simulink model "NL_guidance"  (R2026a)
settings: Solver=ode15s  StopTime=60  MaxStep=0.05  MinStep=1e-8  AbsTol=1e-4
StartFcn:
  | ins_initial_state_xplane;
values from neighbouring files (symbols this model uses):
  C_alt = evalin('base', 'C_alt')    [gui_waypoints.m]    (also in scr_aux_wp.m)
  C_phi = evalin('base', 'C_phi')    [gui_waypoints.m]    (also in scr_aux_wp.m)
  C_theta = evalin('base', 'C_theta')    [gui_waypoints.m]    (also in scr_aux_wp.m)
  C_vel = evalin('base', 'C_vel')    [gui_waypoints.m]    (also in scr_aux_wp.m)
  Kp = evalin('base', 'Kp')    [gui_waypoints.m]    (also in inicializar.m = 0.119; scr_aux_wp.m)
  Kq = evalin('base', 'Kq')    [gui_waypoints.m]    (also in inicializar.m = 0.1; scr_aux_wp.m)
  Kr = evalin('base', 'Kr')    [gui_waypoints.m]    (also in inicializar.m = 0.15; scr_aux_wp.m)
  R_accept = 80    [inicializar.m]    (also in scr_waypoints.m)
  TrimInput = evalin('base', 'TrimInput')    [gui_waypoints.m]    (also in inicializar.m = Ue'; scr_aux_wp.m)
  WPs = [ ... (first row only)    [inicializar.m]
  Xe = evalin('base', 'Xe')    [gui_waypoints.m]    (also in scr_aux_wp.m)
undefined symbols (not defined in the file or in its folder): sensors
libraries: slpidlib x5
settings Model: Creator=anade  LastModifiedBy=julio
settings DataIOCC: SaveState=on

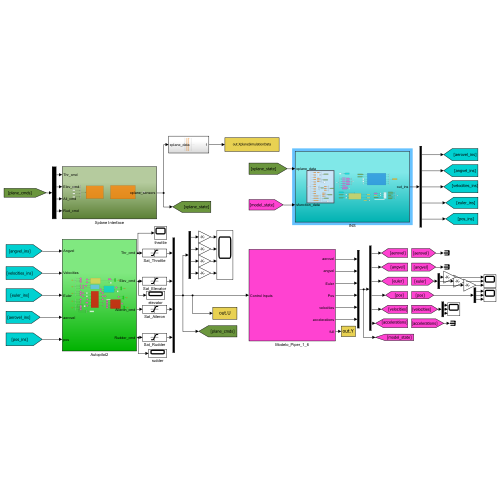
[thumbnail: Simulink's stored preview of the top-level diagram]
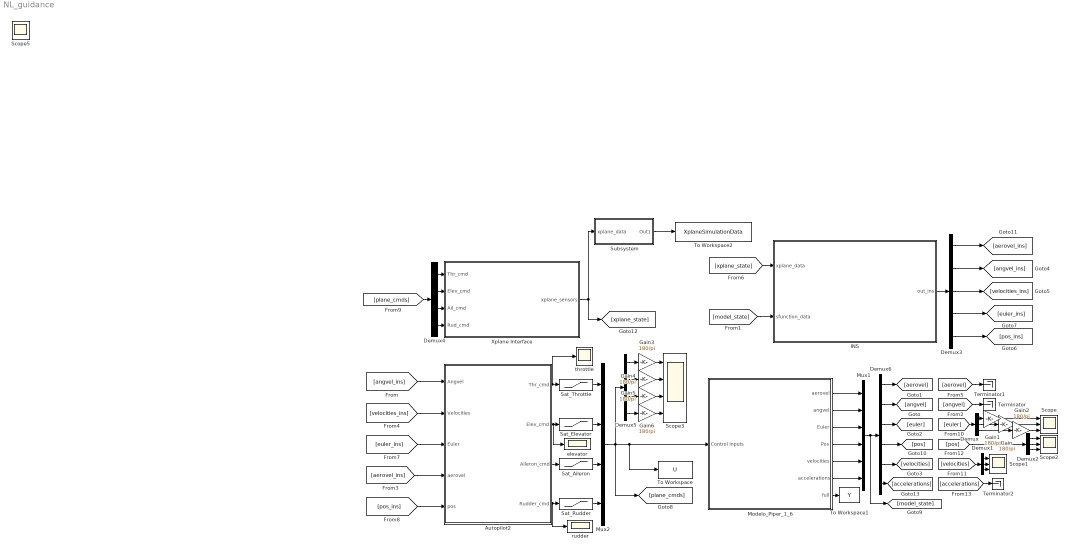
== system NL_guidance ==
  Autopilot2 : Subsystem
  Demux : Demux  Outputs=3
  Demux1 : Demux  Outputs=3
  Demux2 : Demux  Outputs=3
  Demux3 : Demux  Outputs=5
  Demux4 : Demux
  Demux5 : Demux
  Demux6 : Demux  Outputs=6
  Gain{,1..6} (7 alike) : Gain  Gain=180/pi
  INS : Subsystem
  Modelo_Piper_1_6 : Subsystem
  Mux1 : Mux  Inputs=6
  Mux2 : Mux
  Sat_Aileron : Saturate  UpperLimit=0.4363  LowerLimit=-0.4363
  Sat_Elevator : Saturate  UpperLimit=0.4363  LowerLimit=-0.4363
  Sat_Rudder : Saturate  UpperLimit=0.4363  LowerLimit=-0.4363
  Sat_Throttle : Saturate  UpperLimit=1  LowerLimit=0
  Scope : Scope  NumInputPorts=3
      settings: ActiveDisplayYMinimum=-6.98611  ActiveDisplayYMaximum=5.63762
  Scope1 : Scope  NumInputPorts=3
      settings: ActiveDisplayYMinimum=14.85385  ActiveDisplayYMaximum=15.01624
  Scope2 : Scope  NumInputPorts=3
      settings: ActiveDisplayYMinimum=-260.5736  ActiveDisplayYMaximum=2345.16236  DataLoggingVariableName=ScopeData4
  Scope3 : Scope  NumInputPorts=4
      settings: ActiveDisplayYMinimum=27.28743  ActiveDisplayYMaximum=28.20495
  Subsystem : Subsystem
  Terminator : Terminator
  Terminator1 : Terminator
  Terminator2 : Terminator
  To Workspace : ToWorkspace  VariableName=U  SaveFormat=Structure With Time  SampleTime=-1
  To Workspace1 : ToWorkspace  VariableName=Y  SaveFormat=Structure With Time  SampleTime=-1
  To Workspace2 : ToWorkspace  VariableName=XplaneSimulationData  SaveFormat=Structure With Time  SampleTime=-1
  Xplane Interface : Subsystem
  elevator : Scope
      settings: ActiveDisplayYMinimum=-0.5444964451073081  ActiveDisplayYMaximum=0.59983808374051317  DataLoggingVariableName=ScopeData11
  rudder : Scope
      settings: ActiveDisplayYMinimum=-0.082744402354985674  ActiveDisplayYMaximum=0.075589414066673855  DataLoggingVariableName=ScopeData9
  throttle : Scope
      settings: ActiveDisplayYMinimum=-0.079216538751602131  ActiveDisplayYMaximum=0.72681884876441949  DataLoggingVariableName=ScopeData10
  Scope5 : Scope
      settings: ActiveDisplayYMinimum=-10.063291139240507  ActiveDisplayYMaximum=10.936708860759492  DataLoggingVariableName=ScopeData6
  wires:
  Mux2/1 -> [plane_cmds], Demux5/1, To Workspace/1, Modelo_Piper_1_6/1(Control Inputs)
  Modelo_Piper_1_6/7(full) -> To Workspace1/1
  Demux/1 -> Gain1/1
  Demux/2 -> Gain/1
  Demux/3 -> Gain2/1
  Gain/1 -> Scope/2
  Demux1/1 -> Scope1/1
  Demux1/2 -> Scope1/2
  Demux1/3 -> Scope1/3
  Demux2/3 -> Scope2/3
  Demux2/2 -> Scope2/2
  Demux2/1 -> Scope2/1
  [aerovel_ins] -> Autopilot2/4(aerovel)
  Autopilot2/1(Thr_cmd) -> throttle/1, Sat_Throttle/1
  Autopilot2/2(Elev_cmd) -> Sat_Elevator/1, elevator/1
  Autopilot2/3(Aileron_cmd) -> Sat_Aileron/1
  Gain1/1 -> Scope/1
  Gain2/1 -> Scope/3
  Gain3/1 -> Scope3/1
  Gain4/1 -> Scope3/2
  Gain5/1 -> Scope3/3
  Gain6/1 -> Scope3/4
  Sat_Throttle/1 -> Mux2/1
  Sat_Elevator/1 -> Mux2/2
  Sat_Aileron/1 -> Mux2/3
  Sat_Rudder/1 -> Mux2/4
  Demux3/2 -> [angvel_ins]
  Demux3/3 -> [velocities_ins]
  Demux3/4 -> [euler_ins]
  Demux3/5 -> [pos_ins]
  INS/1(out_ins) -> Demux3/1
  [angvel_ins] -> Autopilot2/1(Angvel)
  [velocities_ins] -> Autopilot2/2(Velocities)
  [euler_ins] -> Autopilot2/3(Euler)
  [pos_ins] -> Autopilot2/5(pos)
  [plane_cmds] -> Demux4/1
  Demux4/1 -> Xplane Interface/1(Thr_cmd)
  Demux4/2 -> Xplane Interface/2(Elev_cmd)
  Demux4/3 -> Xplane Interface/3(Ail_cmd)
  Demux4/4 -> Xplane Interface/4(Rud_cmd)
  Demux5/1 -> Gain3/1
  Demux5/2 -> Gain4/1
  Demux5/3 -> Gain5/1
  Demux5/4 -> Gain6/1
  Modelo_Piper_1_6/1(aerovel) -> Mux1/1
  Modelo_Piper_1_6/2(angvel) -> Mux1/2
  Modelo_Piper_1_6/3(Euler) -> Mux1/3
  Modelo_Piper_1_6/4(Pos) -> Mux1/4
  Modelo_Piper_1_6/5(velocities) -> Mux1/5
  Demux6/1 -> [aerovel]
  Demux6/2 -> [angvel]
  Demux6/3 -> [euler]
  Demux6/4 -> [pos]
  Demux6/5 -> [velocities]
  [model_state] -> INS/2(sfunction_data)
  [angvel] -> Terminator/1
  Demux3/1 -> [aerovel_ins]
  [aerovel] -> Terminator1/1
  [pos] -> Demux2/1
  [euler] -> Demux/1
  [velocities] -> Demux1/1
  Xplane Interface/1(xplane_sensors) -> Subsystem/1(xplane_data), [xplane_state]
  [xplane_state] -> INS/1(xplane_data)
  Modelo_Piper_1_6/6(accelerations) -> Mux1/6
  Mux1/1 -> [model_state], Demux6/1
  Demux6/6 -> [accelerations]
  [accelerations] -> Terminator2/1
  Autopilot2/4(Rudder_cmd) -> rudder/1, Sat_Rudder/1
  Subsystem/1(Out1) -> To Workspace2/1

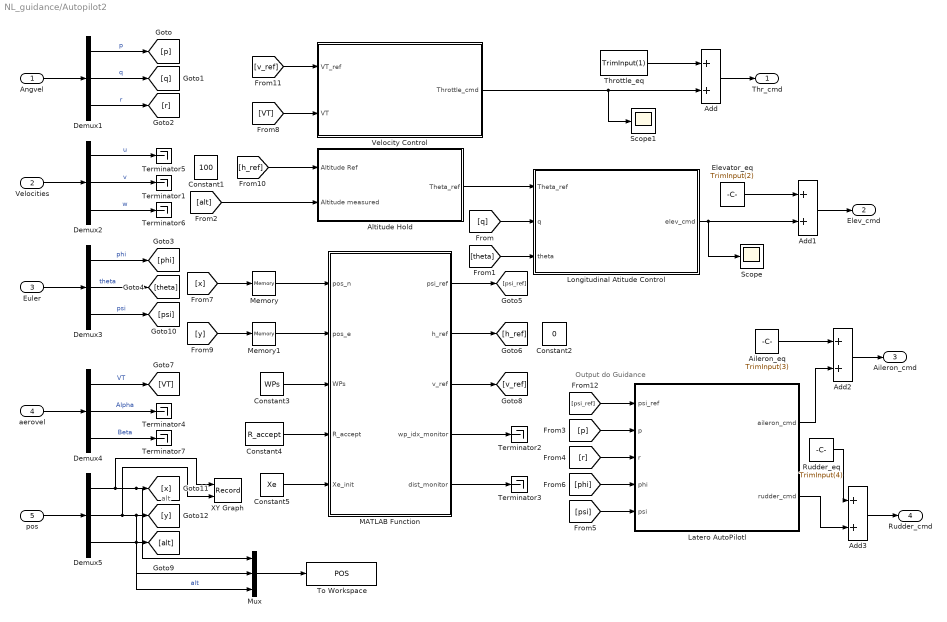
== system NL_guidance/Autopilot2 ==
  note: alt
  note: Output do Guidance
  Angvel : Inport
  Velocities : Inport  Port=2
  Euler : Inport  Port=3
  aerovel : Inport  Port=4
  pos : Inport  Port=5
  Add{,1..3} (4 alike) : Sum
  Aileron_eq : Constant  Value=TrimInput(3)
  Altitude Hold : Subsystem
  Constant1 : Constant  Value=100
  Constant2 : Constant  Value=0
  Constant3 : Constant  Value=WPs
  Constant4 : Constant  Value=R_accept
  Constant5 : Constant  Value=Xe
  Demux{1..5} (5 alike) : Demux  Outputs=3
  Elevator_eq : Constant  Value=TrimInput(2)
  Latero AutoPilotl : Subsystem
  Longitudinal Atitude Control : Subsystem
  MATLAB Function : MATLAB Function  TreatAsAtomicUnit=on
  Memory : Memory  InitialCondition=Xe(10)
  Memory1 : Memory  InitialCondition=Xe(11)
  Mux : Mux  Inputs=3
  Rudder_eq : Constant  Value=TrimInput(4)
  Scope : Scope
      settings: ActiveDisplayYMinimum=-0.12211  ActiveDisplayYMaximum=0.19601
  Scope1 : Scope
      settings: ActiveDisplayYMinimum=-0.14231  ActiveDisplayYMaximum=0.53618  DataLoggingVariableName=ScopeData2
  Terminator{1..7} (7 alike) : Terminator
  Throttle_eq : Constant  Value=TrimInput(1)
  To Workspace : ToWorkspace  VariableName=POS  SaveFormat=Timeseries  SampleTime=-1
  Velocity Control : Subsystem
  XY Graph : Record  NumPorts=2.0  FileSettingsInternal="{\"entries\":[{\"content\":{\"excelSettings\":{\"content\":{},\"type\":\"Streamout.ExcelSettings\"},\"parquetSettings\":{\"content\":{},\"type\":\"Streamout.ParquetSettings\"}},\"type\":\"Streamout.FileSettingStorage\",\"uuid\":\"\"}],\"packageUris\":[\"http:\\/\\/schema.mathworks.com\\/mf0\\/streamout_blocks\\/R2020a\"],\"version\":\"1.0\"}"  FrameSettings=[0, 0]  Layout=[1 1]  SignalsInternal="{\"entries\":[{\"content\":{\"signals\":[{\"content\":{\"blockPath\":[],\"dimensions\":[1],\"domain\":\"\",\"lineColor\":\"#a2142f\",\"plots\":[ 1 ],\"port\":1,\"sid\":[\"\"],\"signalID\":1,\"signalName\":\"Demux5:1\"},\"type\":\"RecordBlkView.Signal\",\"uuid\":\"\"},{\"content\":{\"blockPath\":[],\"dimensions\":[1],\"domain\":\"\",\"lineColor\":\"#139fff\",\"plots\":[ 1 ],\"port\":2,\"sid\":[\"\"],\"signalID\":2,\"signalName\":\"Demux5:2\"},\"type\":\"RecordBlkView.Signal\",\"uuid\":\"\"}]},\"type\":\"RecordBlkView.InputSignals\",\"uuid\":\"\"}],\"packageUris\":[\"http:\\/\\/schema.mathworks.com\\/mf0\\/streamout_blocks\\/R2020a\"],\"version\":\"1.0\"}"  VisualizationBindings="{\"xyplotplugin\":{\"info\":[{\"series\":[{\"bindingParametersList\":[{\"parameter\":\"X-Axis\",\"signalID\":1,\"signalName\":\"Demux5:1\"},{\"parameter\":\"Y-Axis\",\"signalID\":2,\"signalName\":\"Demux5:2\"}],\"seriesID\":0}],\"subplotID\":1}]}}"  CompatibilityTag=XY
  Thr_cmd : Outport
  Elev_cmd : Outport  Port=2
  Aileron_cmd : Outport  Port=3
  Rudder_cmd : Outport  Port=4
  wires:
  Angvel/1 -> Demux1/1
  Velocities/1 -> Demux2/1
  Demux1/1 -> [p]  "p"
  Demux1/2 -> [q]  "q"
  Demux1/3 -> [r]  "r"
  Euler/1 -> Demux3/1
  Demux3/3 -> [psi]  "psi"
  Demux3/1 -> [phi]  "phi"
  Demux3/2 -> [theta]  "theta"
  Demux2/3 -> Terminator6/1  "w"
  Demux2/1 -> Terminator5/1  "u"
  Demux2/2 -> Terminator1/1  "v"
  [theta] -> Longitudinal Atitude Control/3(theta)
  aerovel/1 -> Demux4/1
  Demux4/1 -> [VT]  "VT"
  Demux4/2 -> Terminator4/1  "Alpha"
  Demux4/3 -> Terminator7/1  "Beta"
  Add/1 -> Thr_cmd/1
  Add2/1 -> Aileron_cmd/1
  Add3/1 -> Rudder_cmd/1
  Throttle_eq/1 -> Add/1
  Aileron_eq/1 -> Add2/1
  Rudder_eq/1 -> Add3/1
  [q] -> Longitudinal Atitude Control/2(q)
  Elevator_eq/1 -> Add1/1
  Add1/1 -> Elev_cmd/1
  Longitudinal Atitude Control/1(elev_cmd) -> Add1/2, Scope/1
  [VT] -> Velocity Control/2(VT)
  pos/1 -> Demux5/1
  Demux5/3 -> Mux/3, [alt]  "alt"
  Demux5/2 -> XY Graph/2, Mux/2, [y]
  Latero AutoPilotl/1(aileron_cmd) -> Add2/2
  Latero AutoPilotl/2(rudder_cmd) -> Add3/2
  [p] -> Latero AutoPilotl/2(p)
  [r] -> Latero AutoPilotl/3(r)
  [psi] -> Latero AutoPilotl/5(psi)
  [phi] -> Latero AutoPilotl/4(phi)
  [v_ref] -> Velocity Control/1(VT_ref)
  Velocity Control/1(Throttle_cmd) -> Scope1/1, Add/2
  Altitude Hold/1(Theta_ref) -> Longitudinal Atitude Control/1(Theta_ref)
  [alt] -> Altitude Hold/2(Altitude measured)
  Constant4/1 -> MATLAB Function/4(R_accept)
  Constant3/1 -> MATLAB Function/3(WPs)
  MATLAB Function/2(h_ref) -> [h_ref]
  Constant5/1 -> MATLAB Function/5(Xe_init)
  MATLAB Function/1(psi_ref) -> [psi_ref]
  MATLAB Function/3(v_ref) -> [v_ref]
  [h_ref] -> Altitude Hold/1(Altitude Ref)
  [x] -> Memory/1
  Memory/1 -> MATLAB Function/1(pos_n)
  [y] -> Memory1/1
  Memory1/1 -> MATLAB Function/2(pos_e)
  [psi_ref] -> Latero AutoPilotl/1(psi_ref)
  Demux5/1 -> XY Graph/1, Mux/1, [x]
  MATLAB Function/4(wp_idx_monitor) -> Terminator2/1
  MATLAB Function/5(dist_monitor) -> Terminator3/1
  Mux/1 -> To Workspace/1

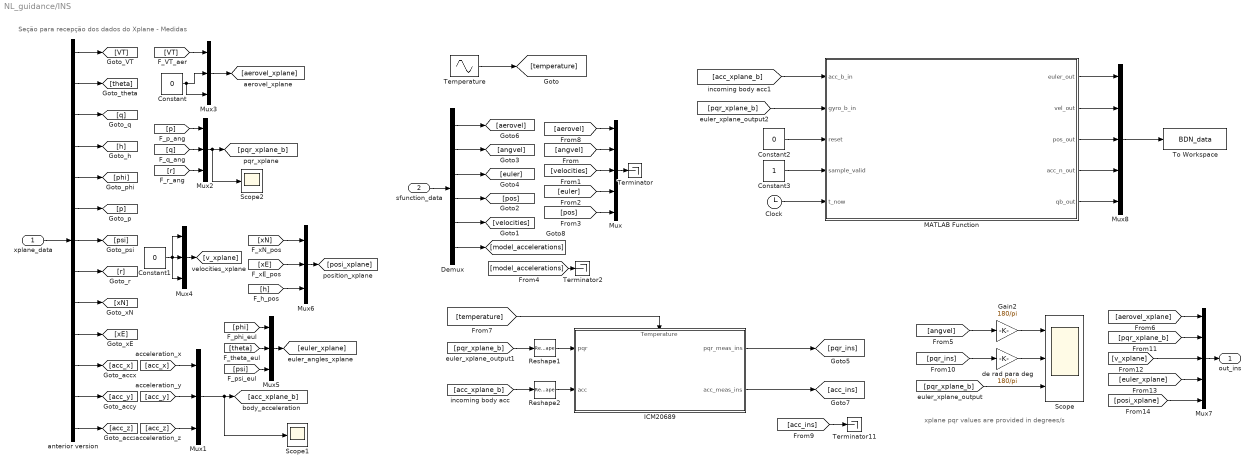
== system NL_guidance/INS ==
  note: xplane pqr values are provided in degrees/s
  note: Seção para recepção dos dados do Xplane - Medidas
  xplane_data : Inport
  sfunction_data : Inport  Port=2
  Clock : Clock
  Constant : Constant  Value=0
  Constant1 : Constant  Value=0
  Constant2 : Constant  Value=0
  Constant3 : Constant
  Demux : Demux  Outputs=6
  Gain2 : Gain  Gain=180/pi
  ICM20689 : Subsystem
      settings: PortSchema="{\"entries\":[{\"content\":{\"sides\":[{\"content\":{\"connectorIds\":[\"In1\",\"In2\"]},\"type\":\"ConnectorPlacement.EquallySpacedRectSide\",\"uuid\":\"9b78a035-9d4a-478e-9dc9-dc0bea5c931a\"},{\"content\":{\"connectorIds\":[\"Out1\",\"Out2\"],\"side\":\"RIGHT\"},\"type\":\"ConnectorPlacement.EquallySpacedRectSide\",\"uuid\":\"e21d77f8-fafe-45cf-b395-99fef016bd99\"},{\"content\":{\"connectorIds\":[\"In3\"],\"side\":\"TOP\"},\"type\":\"ConnectorPlacement.EquallySpacedRectSide\",\"uuid\":\"145a04c5-db60-4d84-a30a-895cdbce0dc0\"},{\"content\":{\"side\":\"BOTTOM\"},\"type\":\"ConnectorPlacement.EquallySpacedRectSide\",\"uuid\":\"826403f1-12d1-4d95-a630-f2fb059454f4\"}]},\"type\":\"ConnectorPlacement.EquallySpacedConnector\",\"uuid\":\"784d3b4a-97ce-487c-94bc-bef96ce83330\"}],\"packageUris\":[\"http://schema.mathworks.com/mf0/Connector/R2020b\"],\"version\":\"1.0\"}"
  MATLAB Function : MATLAB Function  TreatAsAtomicUnit=on
  Mux : Mux  Inputs=5
  Mux{1..6} (6 alike) : Mux  Inputs=3
  Mux7 : Mux  Inputs=5
  Mux8 : Mux  Inputs=5
  Reshape1 : Reshape  OutputDimensionality=Customize  OutputDimensions=[3 1]
  Reshape2 : Reshape  OutputDimensionality=Customize  OutputDimensions=[3 1]
  Scope : Scope  NumInputPorts=3
      settings: ActiveDisplayYMinimum=-72.109974321160792  ActiveDisplayYMaximum=81.22468249036686
  Scope1 : Scope
      settings: ActiveDisplayYMinimum=-16.174539597742694  ActiveDisplayYMaximum=12.212616009640644  DataLoggingVariableName=ScopeData7
  Scope2 : Scope
      settings: DataLoggingVariableName=ScopeData8
  Temperature : Sin  Amplitude=10  Bias=25  Frequency=2*pi*0.01  SampleTime=0
  Terminator : Terminator
  Terminator11 : Terminator
  Terminator2 : Terminator
  To Workspace : ToWorkspace  VariableName=BDN_data  SaveFormat=Structure With Time  SampleTime=-1
  anterior version : Demux  Outputs=13
  de rad para deg : Gain  Gain=180/pi
  out_ins : Outport
  wires:
  Reshape1/1 -> ICM20689/1(pqr)
  sfunction_data/1 -> Demux/1
  Demux/2 -> [angvel]
  [velocities] -> Mux/3
  [euler] -> Mux/4
  [pos] -> Mux/5
  de rad para deg/1 -> Scope/2
  ICM20689/1(pqr_meas_ins) -> [pqr_ins]
  [angvel] -> Mux/2
  Temperature/1 -> [temperature]
  [temperature] -> ICM20689/3(Temperature)
  Gain2/1 -> Scope/1
  [angvel] -> Gain2/1
  xplane_data/1 -> anterior version/1
  anterior version/1 -> [VT]
  anterior version/6 -> [p]
  anterior version/9 -> [xN]
  anterior version/3 -> [q]
  anterior version/8 -> [r]
  anterior version/5 -> [phi]
  anterior version/10 -> [xE]
  anterior version/2 -> [theta]
  anterior version/7 -> [psi]
  anterior version/4 -> [h]
  anterior version/11 -> [acc_x]
  anterior version/12 -> [acc_y]
  anterior version/13 -> [acc_z]
  [VT] -> Mux3/1
  [p] -> Mux2/1
  [r] -> Mux2/3
  [acc_x] -> Mux1/1
  [acc_y] -> Mux1/2
  [acc_z] -> Mux1/3
  Mux1/1 -> Scope1/1, [acc_xplane_b]
  ICM20689/2(acc_meas_ins) -> [acc_ins]
  [acc_ins] -> Terminator11/1
  Mux2/1 -> Scope2/1, [pqr_xplane_b]
  [pqr_xplane_b] -> Scope/3
  [pqr_ins] -> de rad para deg/1
  [q] -> Mux2/2
  Demux/1 -> [aerovel]
  [aerovel] -> Mux/1
  Demux/5 -> [velocities]
  Demux/4 -> [pos]
  Demux/3 -> [euler]
  [pqr_xplane_b] -> Reshape1/1
  Reshape2/1 -> ICM20689/2(acc)
  [acc_xplane_b] -> Reshape2/1
  Demux/6 -> [model_accelerations]
  [model_accelerations] -> Terminator2/1
  Constant/1 -> Mux3/3, Mux3/2
  Mux3/1 -> [aerovel_xplane]
  Constant1/1 -> Mux4/3, Mux4/1, Mux4/2
  Mux4/1 -> [v_xplane]
  Mux5/1 -> [euler_xplane]
  [phi] -> Mux5/1
  [theta] -> Mux5/2
  [psi] -> Mux5/3
  [xN] -> Mux6/1
  [xE] -> Mux6/2
  [h] -> Mux6/3
  Mux6/1 -> [posi_xplane]
  [aerovel_xplane] -> Mux7/1
  [pqr_xplane_b] -> Mux7/2
  [v_xplane] -> Mux7/3
  [euler_xplane] -> Mux7/4
  [posi_xplane] -> Mux7/5
  Mux/1 -> Terminator/1
  Mux7/1 -> out_ins/1
  [acc_xplane_b] -> MATLAB Function/1(acc_b_in)
  [pqr_xplane_b] -> MATLAB Function/2(gyro_b_in)
  Constant2/1 -> MATLAB Function/3(reset)
  Constant3/1 -> MATLAB Function/4(sample_valid)
  Clock/1 -> MATLAB Function/5(t_now)
  MATLAB Function/1(euler_out) -> Mux8/1
  MATLAB Function/2(vel_out) -> Mux8/2
  MATLAB Function/3(pos_out) -> Mux8/3
  MATLAB Function/4(acc_n_out) -> Mux8/4
  MATLAB Function/5(qb_out) -> Mux8/5
  Mux8/1 -> To Workspace/1

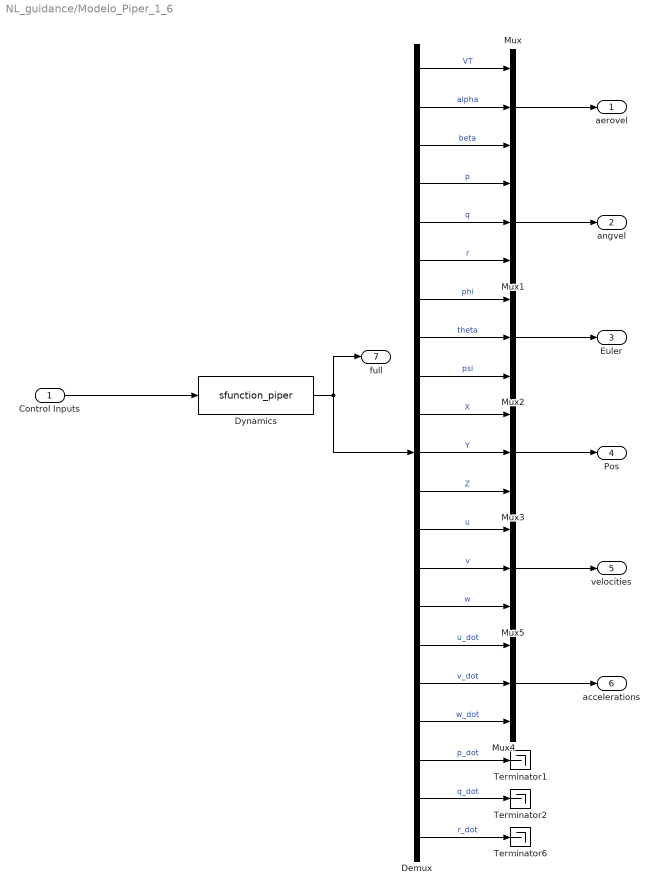
== system NL_guidance/Modelo_Piper_1_6 ==
  Control Inputs : Inport
  Demux : Demux  Outputs=21
  Dynamics : S-Function  FunctionName=sfunction_piper  Parameters=par_gen,par_aero,par_prop, Xe  SFunctionDeploymentMode=off  EnableBusSupport=off
  Mux{,1..5} (6 alike) : Mux  Inputs=3
  Terminator1 : Terminator
  Terminator2 : Terminator
  Terminator6 : Terminator
  aerovel : Outport
  angvel : Outport  Port=2
  Euler : Outport  Port=3
  Pos : Outport  Port=4
  velocities : Outport  Port=5
  accelerations : Outport  Port=6
  full : Outport  Port=7
  wires:
  Control Inputs/1 -> Dynamics/1
  Dynamics/1 -> full/1, Demux/1
  Demux/1 -> Mux/1  "VT"
  Demux/2 -> Mux/2  "alpha"
  Demux/3 -> Mux/3  "beta"
  Mux/1 -> aerovel/1
  Demux/6 -> Mux1/3  "r"
  Demux/4 -> Mux1/1  "p"
  Mux1/1 -> angvel/1
  Demux/5 -> Mux1/2  "q"
  Mux2/1 -> Euler/1
  Demux/9 -> Mux2/3  "psi"
  Demux/7 -> Mux2/1  "phi"
  Demux/8 -> Mux2/2  "theta"
  Demux/11 -> Mux3/2  "Y"
  Demux/10 -> Mux3/1  "X"
  Demux/12 -> Mux3/3  "Z"
  Mux3/1 -> Pos/1
  Demux/14 -> Mux5/2  "v"
  Demux/15 -> Mux5/3  "w"
  Demux/17 -> Mux4/2  "v_dot"
  Demux/18 -> Mux4/3  "w_dot"
  Demux/16 -> Mux4/1  "u_dot"
  Demux/19 -> Terminator1/1  "p_dot"
  Demux/20 -> Terminator2/1  "q_dot"
  Demux/21 -> Terminator6/1  "r_dot"
  Demux/13 -> Mux5/1  "u"
  Mux5/1 -> velocities/1
  Mux4/1 -> accelerations/1

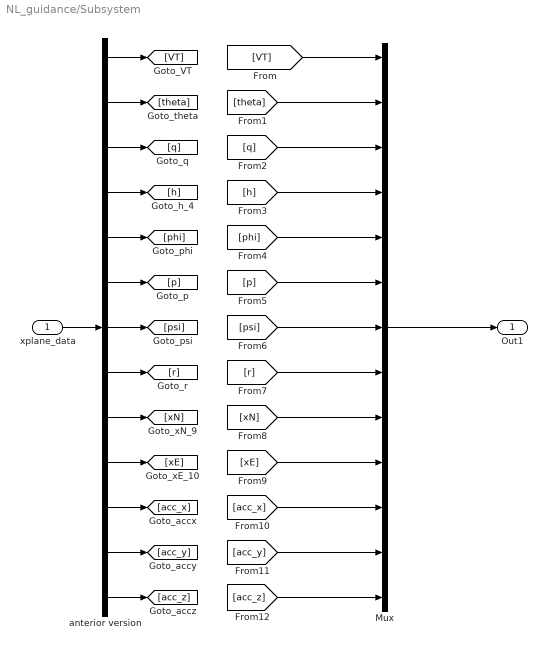
== system NL_guidance/Subsystem ==
  xplane_data : Inport
  Mux : Mux  Inputs=13
  anterior version : Demux  Outputs=13
  Out1 : Outport
  wires:
  anterior version/3 -> [q]
  anterior version/8 -> [r]
  anterior version/4 -> [h]
  anterior version/2 -> [theta]
  anterior version/6 -> [p]
  anterior version/1 -> [VT]
  xplane_data/1 -> anterior version/1
  anterior version/9 -> [xN]
  anterior version/12 -> [acc_y]
  anterior version/11 -> [acc_x]
  anterior version/13 -> [acc_z]
  anterior version/10 -> [xE]
  anterior version/7 -> [psi]
  anterior version/5 -> [phi]
  [VT] -> Mux/1
  [theta] -> Mux/2
  [q] -> Mux/3
  [h] -> Mux/4
  [phi] -> Mux/5
  [p] -> Mux/6
  [psi] -> Mux/7
  [r] -> Mux/8
  [xN] -> Mux/9
  [xE] -> Mux/10
  [acc_x] -> Mux/11
  [acc_y] -> Mux/12
  [acc_z] -> Mux/13
  Mux/1 -> Out1/1

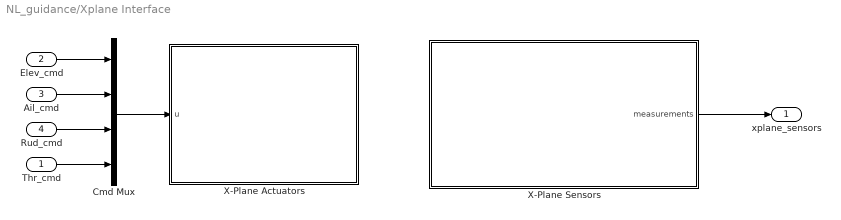
== system NL_guidance/Xplane Interface ==
  Thr_cmd : Inport
  Elev_cmd : Inport  Port=2
  Ail_cmd : Inport  Port=3
  Rud_cmd : Inport  Port=4
  Cmd Mux : Mux
  X-Plane Actuators : MATLAB Function  TreatAsAtomicUnit=on
  X-Plane Sensors : MATLAB Function  TreatAsAtomicUnit=on
  xplane_sensors : Outport
  wires:
  Cmd Mux/1 -> X-Plane Actuators/1(u)
  X-Plane Sensors/1(measurements) -> xplane_sensors/1
  Elev_cmd/1 -> Cmd Mux/1
  Ail_cmd/1 -> Cmd Mux/2
  Rud_cmd/1 -> Cmd Mux/3
  Thr_cmd/1 -> Cmd Mux/4

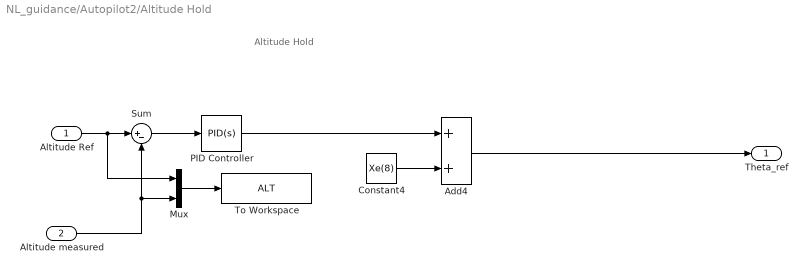
== system NL_guidance/Autopilot2/Altitude Hold ==
  note: Altitude Hold
  Altitude Ref : Inport
  Altitude measured : Inport  Port=2
  Add4 : Sum
  Constant4 : Constant  Value=Xe(8)
  Mux : Mux  Inputs=2
  PID Controller : slpidlib/PID Controller  Controller=PID  Form=Parallel  TimeDomain=Continuous-time  UseExternalTs=off  SampleTime=-1  IntegratorMethod=Forward Euler  FilterMethod=Forward Euler  ControllerParametersSource=internal  P=C_alt.Kp  I=C_alt.Ki  UseKiTs=off  D=C_alt.Kd  UseExternalDerivativeSource=off  N=C_alt.N  UseFilter=on  TunerSelectOption=Transfer Function Based (PID Tuner App)  InitialConditionSource=internal  InitialConditionForIntegrator=0  InitialConditionForFilter=0  DifferentiatorICPrevScaledInput=0  ExternalReset=none  TrackingMode=off  Kt=1  LimitOutput=on  SatLimitsSource=internal  UpperSaturationLimit=0.26  LowerSaturationLimit=-0.17  LinearizeAsGain=on  AntiWindupMode=back-calculation  Kb=1  LimitIntegrator=off  UpperIntegratorSaturationLimit=inf  LowerIntegratorSaturationLimit=-inf  POutMin=[]  POutMax=[]  IOutMin=[]  IOutMax=[]  DOutMin=[]  DOutMax=[]  NOutMin=[]  NOutMax=[]  SumOutMin=[]  SumOutMax=[]  SaturationOutMin=[]  SaturationOutMax=[]  PParamMin=[]  PParamMax=[]  IParamMin=[]  IParamMax=[]  DParamMin=[]  DParamMax=[]  NParamMin=[]  NParamMax=[]  KbParamMin=[]  KbParamMax=[]  KtParamMin=[]  KtParamMax=[]  KbOutMin=[]  KbOutMax=[]  KtOutMin=[]  KtOutMax=[]  IntegratorOutMin=[]  IntegratorOutMax=[]  FilterOutMin=[]  FilterOutMax=[]  SumI1OutMin=[]  SumI1OutMax=[]  SumI2OutMin=[]  SumI2OutMax=[]  SumI3OutMin=[]  SumI3OutMax=[]  SumI4OutMin=[]  SumI4OutMax=[]  SumDOutMin=[]  SumDOutMax=[]  DifferentiatorOutMin=[]  DifferentiatorOutMax=[]  FilterDiffOutCoefMin=[]  FilterDiffOutCoefMax=[]  ReciprocalOutMin=[]  ReciprocalOutMax=[]  SumDenOutMin=[]  SumDenOutMax=[]  SumNumOutMin=[]  SumNumOutMax=[]  DivideOutMin=[]  DivideOutMax=[]  UdiffTsProdOutMin=[]  UdiffTsProdOutMax=[]  NTsProdOutMin=[]  NTsProdOutMax=[]  UintegralTsProdOutMin=[]  UintegralTsProdOutMax=[]  UngainTsProdOutMin=[]  UngainTsProdOutMax=[]  ClampingZeroOutDataTypeStr=Inherit: Inherit via back propagation  ClampingZeroOutMin=[]  ClampingZeroOutMax=[]  FilterDenConstantOutDataTypeStr=Inherit: Inherit via back propagation  FilterDenConstantOutMin=[]  FilterDenConstantOutMax=[]  PCopyOutDataTypeStr=Inherit: Inherit via back propagation  PCopyOutMin=[]  PCopyOutMax=[]  NCopyOutDataTypeStr=Inherit: Inherit via back propagation  NCopyOutMin=[]  NCopyOutMax=[]  IntegratorContinuousStateAttributes=''  IntegratorStateMustResolveToSignalObject=off  IntegratorRTWStateStorageClass=Auto  FilterContinuousStateAttributes=''  FilterStateMustResolveToSignalObject=off  FilterRTWStateStorageClass=Auto  ParallelPVariant=InternalParameters  IdealPVariant=Disabled  IVariant=InternalParameters  DVariant=InternalParameters  IntegratorVariant=Continuous  SatVariant=Enabled  AWVariant=BackCalculation  PCopyVariant=Disabled  TRVariant=Disabled  FdbkBlocksVariant=Forward  IdealPFdbkVariant=Disabled  SatFdbkVariant=Disabled  DerivativeFilterVariant=ContFilter  NVariant=InternalParameters  NCopyVariant=Disabled  FilterICVariant=InternalICsFilter  IntegratorICVariant=InternalICs  ExternalResetVariant=Disabled  TRSumVariant=Passthrough  SumFdbkVariant=Disabled  SumVariant=Sum_PID  TsampFilterVariant=InternalTs  TsampNgainVariant=Passthrough  TsampIntegralVariant=Disabled_SignalSpec  ExternalSaturationOutDataTypeStr=Inherit: Same as second input  DerivativeSourceVariant=ErrorSignal  PreIntVariant=InternalPreInt
  Sum : Sum  Inputs=|+-
  To Workspace : ToWorkspace  VariableName=ALT  SaveFormat=Timeseries  SampleTime=-1
  Theta_ref : Outport
  wires:
  Altitude Ref/1 -> Mux/1, Sum/1
  PID Controller/1 -> Add4/1
  Add4/1 -> Theta_ref/1
  Constant4/1 -> Add4/2
  Sum/1 -> PID Controller/1
  Altitude measured/1 -> Mux/2, Sum/2
  Mux/1 -> To Workspace/1

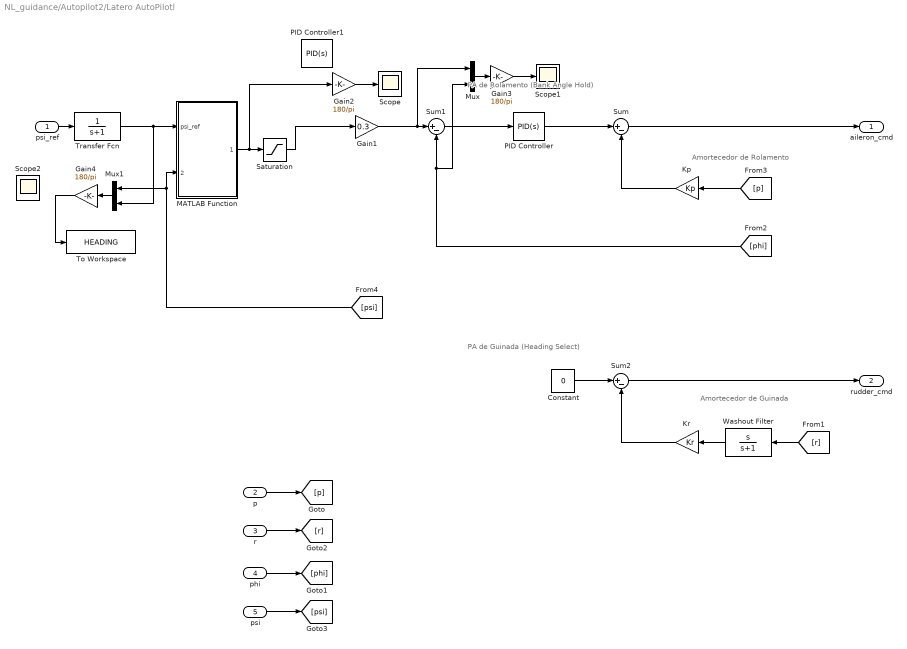
== system NL_guidance/Autopilot2/Latero AutoPilotl ==
  note: PA de Rolamento (Bank Angle Hold)
  note: Amortecedor de Rolamento
  note: Amortecedor de Guinada
  note: PA de Guinada (Heading Select)
  psi_ref : Inport
  p : Inport  Port=2
  r : Inport  Port=3
  phi : Inport  Port=4
  psi : Inport  Port=5
  Constant : Constant  Value=0
  Gain1 : Gain  Gain=0.3
  Gain2 : Gain  Gain=180/pi
  Gain3 : Gain  Gain=180/pi
  Gain4 : Gain  Gain=180/pi
  Kp : Gain  Gain=Kp
  Kr : Gain  Gain=Kr
  MATLAB Function : MATLAB Function  TreatAsAtomicUnit=on
  Mux : Mux  Inputs=2
  Mux1 : Mux  Inputs=2
  PID Controller : slpidlib/PID Controller  Controller=PID  Form=Parallel  TimeDomain=Continuous-time  UseExternalTs=off  SampleTime=-1  IntegratorMethod=Forward Euler  FilterMethod=Forward Euler  ControllerParametersSource=internal  P=C_phi.Kp  I=C_phi.Ki  UseKiTs=off  D=C_phi.Kd  UseExternalDerivativeSource=off  N=C_phi.N  UseFilter=on  TunerSelectOption=Transfer Function Based (PID Tuner App)  InitialConditionSource=internal  InitialConditionForIntegrator=0  InitialConditionForFilter=0  DifferentiatorICPrevScaledInput=0  ExternalReset=none  TrackingMode=off  Kt=1  LimitOutput=on  SatLimitsSource=internal  UpperSaturationLimit=0.43  LowerSaturationLimit=-0.43  LinearizeAsGain=on  AntiWindupMode=back-calculation  Kb=1  LimitIntegrator=off  UpperIntegratorSaturationLimit=inf  LowerIntegratorSaturationLimit=-inf  POutMin=[]  POutMax=[]  IOutMin=[]  IOutMax=[]  DOutMin=[]  DOutMax=[]  NOutMin=[]  NOutMax=[]  SumOutMin=[]  SumOutMax=[]  SaturationOutMin=[]  SaturationOutMax=[]  PParamMin=[]  PParamMax=[]  IParamMin=[]  IParamMax=[]  DParamMin=[]  DParamMax=[]  NParamMin=[]  NParamMax=[]  KbParamMin=[]  KbParamMax=[]  KtParamMin=[]  KtParamMax=[]  KbOutMin=[]  KbOutMax=[]  KtOutMin=[]  KtOutMax=[]  IntegratorOutMin=[]  IntegratorOutMax=[]  FilterOutMin=[]  FilterOutMax=[]  SumI1OutMin=[]  SumI1OutMax=[]  SumI2OutMin=[]  SumI2OutMax=[]  SumI3OutMin=[]  SumI3OutMax=[]  SumI4OutMin=[]  SumI4OutMax=[]  SumDOutMin=[]  SumDOutMax=[]  DifferentiatorOutMin=[]  DifferentiatorOutMax=[]  FilterDiffOutCoefMin=[]  FilterDiffOutCoefMax=[]  ReciprocalOutMin=[]  ReciprocalOutMax=[]  SumDenOutMin=[]  SumDenOutMax=[]  SumNumOutMin=[]  SumNumOutMax=[]  DivideOutMin=[]  DivideOutMax=[]  UdiffTsProdOutMin=[]  UdiffTsProdOutMax=[]  NTsProdOutMin=[]  NTsProdOutMax=[]  UintegralTsProdOutMin=[]  UintegralTsProdOutMax=[]  UngainTsProdOutMin=[]  UngainTsProdOutMax=[]  ClampingZeroOutDataTypeStr=Inherit: Inherit via back propagation  ClampingZeroOutMin=[]  ClampingZeroOutMax=[]  FilterDenConstantOutDataTypeStr=Inherit: Inherit via back propagation  FilterDenConstantOutMin=[]  FilterDenConstantOutMax=[]  PCopyOutDataTypeStr=Inherit: Inherit via back propagation  PCopyOutMin=[]  PCopyOutMax=[]  NCopyOutDataTypeStr=Inherit: Inherit via back propagation  NCopyOutMin=[]  NCopyOutMax=[]  IntegratorContinuousStateAttributes=''  IntegratorStateMustResolveToSignalObject=off  IntegratorRTWStateStorageClass=Auto  FilterContinuousStateAttributes=''  FilterStateMustResolveToSignalObject=off  FilterRTWStateStorageClass=Auto  ParallelPVariant=InternalParameters  IdealPVariant=Disabled  IVariant=InternalParameters  DVariant=InternalParameters  IntegratorVariant=Continuous  SatVariant=Enabled  AWVariant=BackCalculation  PCopyVariant=Disabled  TRVariant=Disabled  FdbkBlocksVariant=Forward  IdealPFdbkVariant=Disabled  SatFdbkVariant=Disabled  DerivativeFilterVariant=ContFilter  NVariant=InternalParameters  NCopyVariant=Disabled  FilterICVariant=InternalICsFilter  IntegratorICVariant=InternalICs  ExternalResetVariant=Disabled  TRSumVariant=Passthrough  SumFdbkVariant=Disabled  SumVariant=Sum_PID  TsampFilterVariant=InternalTs  TsampNgainVariant=Passthrough  TsampIntegralVariant=Disabled_SignalSpec  ExternalSaturationOutDataTypeStr=Inherit: Same as second input  DerivativeSourceVariant=ErrorSignal  PreIntVariant=InternalPreInt
  PID Controller1 : slpidlib/PID Controller  Controller=PID  Form=Parallel  TimeDomain=Continuous-time  UseExternalTs=off  SampleTime=-1  IntegratorMethod=Forward Euler  FilterMethod=Forward Euler  ControllerParametersSource=internal  P=2.5  I=0  UseKiTs=off  D=0  UseExternalDerivativeSource=off  N=100  UseFilter=on  TunerSelectOption=Transfer Function Based (PID Tuner App)  InitialConditionSource=internal  InitialConditionForIntegrator=0  InitialConditionForFilter=0  DifferentiatorICPrevScaledInput=0  ExternalReset=none  TrackingMode=off  Kt=1  LimitOutput=off  SatLimitsSource=internal  UpperSaturationLimit=inf  LowerSaturationLimit=-inf  LinearizeAsGain=on  AntiWindupMode=none  Kb=1  LimitIntegrator=off  UpperIntegratorSaturationLimit=inf  LowerIntegratorSaturationLimit=-inf  POutMin=[]  POutMax=[]  IOutMin=[]  IOutMax=[]  DOutMin=[]  DOutMax=[]  NOutMin=[]  NOutMax=[]  SumOutMin=[]  SumOutMax=[]  SaturationOutMin=[]  SaturationOutMax=[]  PParamMin=[]  PParamMax=[]  IParamMin=[]  IParamMax=[]  DParamMin=[]  DParamMax=[]  NParamMin=[]  NParamMax=[]  KbParamMin=[]  KbParamMax=[]  KtParamMin=[]  KtParamMax=[]  KbOutMin=[]  KbOutMax=[]  KtOutMin=[]  KtOutMax=[]  IntegratorOutMin=[]  IntegratorOutMax=[]  FilterOutMin=[]  FilterOutMax=[]  SumI1OutMin=[]  SumI1OutMax=[]  SumI2OutMin=[]  SumI2OutMax=[]  SumI3OutMin=[]  SumI3OutMax=[]  SumI4OutMin=[]  SumI4OutMax=[]  SumDOutMin=[]  SumDOutMax=[]  DifferentiatorOutMin=[]  DifferentiatorOutMax=[]  FilterDiffOutCoefMin=[]  FilterDiffOutCoefMax=[]  ReciprocalOutMin=[]  ReciprocalOutMax=[]  SumDenOutMin=[]  SumDenOutMax=[]  SumNumOutMin=[]  SumNumOutMax=[]  DivideOutMin=[]  DivideOutMax=[]  UdiffTsProdOutMin=[]  UdiffTsProdOutMax=[]  NTsProdOutMin=[]  NTsProdOutMax=[]  UintegralTsProdOutMin=[]  UintegralTsProdOutMax=[]  UngainTsProdOutMin=[]  UngainTsProdOutMax=[]  ClampingZeroOutDataTypeStr=Inherit: Inherit via back propagation  ClampingZeroOutMin=[]  ClampingZeroOutMax=[]  FilterDenConstantOutDataTypeStr=Inherit: Inherit via back propagation  FilterDenConstantOutMin=[]  FilterDenConstantOutMax=[]  PCopyOutDataTypeStr=Inherit: Inherit via back propagation  PCopyOutMin=[]  PCopyOutMax=[]  NCopyOutDataTypeStr=Inherit: Inherit via back propagation  NCopyOutMin=[]  NCopyOutMax=[]  IntegratorContinuousStateAttributes=''  IntegratorStateMustResolveToSignalObject=off  IntegratorRTWStateStorageClass=Auto  FilterContinuousStateAttributes=''  FilterStateMustResolveToSignalObject=off  FilterRTWStateStorageClass=Auto  ParallelPVariant=InternalParameters  IdealPVariant=Disabled  IVariant=InternalParameters  DVariant=InternalParameters  IntegratorVariant=Continuous  SatVariant=Disabled  AWVariant=Passthrough  PCopyVariant=Disabled  TRVariant=Disabled  FdbkBlocksVariant=Forward  IdealPFdbkVariant=Disabled  SatFdbkVariant=Disabled  DerivativeFilterVariant=ContFilter  NVariant=InternalParameters  NCopyVariant=Disabled  FilterICVariant=InternalICsFilter  IntegratorICVariant=InternalICs  ExternalResetVariant=Disabled  TRSumVariant=Passthrough  SumFdbkVariant=Disabled  SumVariant=Sum_PID  TsampFilterVariant=InternalTs  TsampNgainVariant=Passthrough  TsampIntegralVariant=Disabled_SignalSpec  ExternalSaturationOutDataTypeStr=Inherit: Same as second input  DerivativeSourceVariant=ErrorSignal  PreIntVariant=InternalPreInt
  Saturation : Saturate  UpperLimit=1.0  LowerLimit=-1.0
  Scope : Scope
      settings: ActiveDisplayYMinimum=-3.05499  ActiveDisplayYMaximum=27.49487  DataLoggingVariableName=ScopeData3
  Scope1 : Scope
      settings: ActiveDisplayYMinimum=-0.54177  ActiveDisplayYMaximum=4.86179  DataLoggingVariableName=ScopeData4
  Scope2 : Scope
      settings: ActiveDisplayYMinimum=-1  ActiveDisplayYMaximum=1  DataLoggingVariableName=ScopeData5
  Sum : Sum  Inputs=|+-
  Sum1 : Sum  Inputs=|+-
  Sum2 : Sum  Inputs=|+-
  To Workspace : ToWorkspace  VariableName=HEADING  SampleTime=-1
  Transfer Fcn : TransferFcn  Denominator=[1 1]
  Washout Filter : TransferFcn  Numerator=[1 0]  Denominator=[1 1]
  aileron_cmd : Outport
  rudder_cmd : Outport  Port=2
  wires:
  Sum/1 -> aileron_cmd/1
  [p] -> Kp/1
  [phi] -> Mux/2, Sum1/2
  Kp/1 -> Sum/2
  PID Controller/1 -> Sum/1
  p/1 -> [p]
  [r] -> Washout Filter/1
  Kr/1 -> Sum2/2
  r/1 -> [r]
  Washout Filter/1 -> Kr/1
  phi/1 -> [phi]
  psi/1 -> [psi]
  Sum2/1 -> rudder_cmd/1
  Constant/1 -> Sum2/1
  Gain1/1 -> Mux/1, Sum1/1
  psi_ref/1 -> Transfer Fcn/1
  [psi] -> Mux1/1, MATLAB Function/2(psi_atual)
  MATLAB Function/1(erro_psi) -> Gain2/1, Saturation/1
  Gain2/1 -> Scope/1
  Saturation/1 -> Gain1/1
  Gain3/1 -> Scope1/1
  Sum1/1 -> PID Controller/1
  Mux/1 -> Gain3/1
  Mux1/1 -> Gain4/1
  Transfer Fcn/1 -> Mux1/2, MATLAB Function/1(psi_ref)
  Gain4/1 -> To Workspace/1

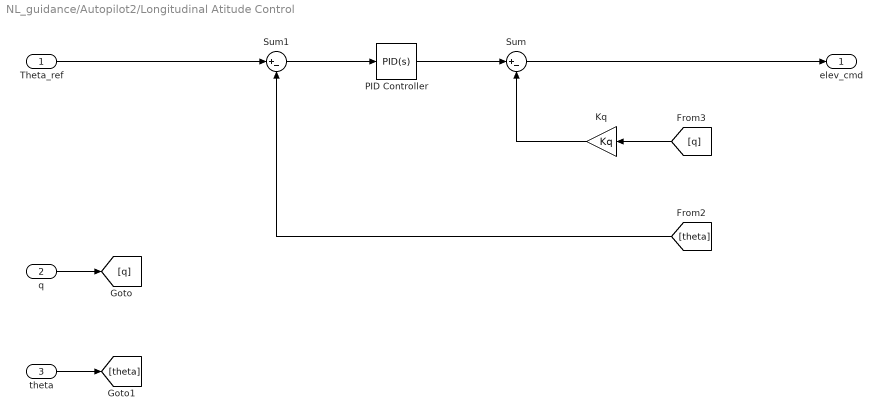
== system NL_guidance/Autopilot2/Longitudinal Atitude Control ==
  Theta_ref : Inport
  q : Inport  Port=2
  theta : Inport  Port=3
  Kq : Gain  Gain=Kq
  PID Controller : slpidlib/PID Controller  Controller=PID  Form=Parallel  TimeDomain=Continuous-time  UseExternalTs=off  SampleTime=-1  IntegratorMethod=Forward Euler  FilterMethod=Forward Euler  ControllerParametersSource=internal  P=C_theta.Kp  I=C_theta.Ki  UseKiTs=off  D=C_theta.Kd  UseExternalDerivativeSource=off  N=C_theta.N  UseFilter=on  TunerSelectOption=Transfer Function Based (PID Tuner App)  InitialConditionSource=internal  InitialConditionForIntegrator=0  InitialConditionForFilter=0  DifferentiatorICPrevScaledInput=0  ExternalReset=none  TrackingMode=off  Kt=1  LimitOutput=on  SatLimitsSource=internal  UpperSaturationLimit=0.4363  LowerSaturationLimit=-0.4363  LinearizeAsGain=on  AntiWindupMode=back-calculation  Kb=1  LimitIntegrator=off  UpperIntegratorSaturationLimit=inf  LowerIntegratorSaturationLimit=-inf  POutMin=[]  POutMax=[]  IOutMin=[]  IOutMax=[]  DOutMin=[]  DOutMax=[]  NOutMin=[]  NOutMax=[]  SumOutMin=[]  SumOutMax=[]  SaturationOutMin=[]  SaturationOutMax=[]  PParamMin=[]  PParamMax=[]  IParamMin=[]  IParamMax=[]  DParamMin=[]  DParamMax=[]  NParamMin=[]  NParamMax=[]  KbParamMin=[]  KbParamMax=[]  KtParamMin=[]  KtParamMax=[]  KbOutMin=[]  KbOutMax=[]  KtOutMin=[]  KtOutMax=[]  IntegratorOutMin=[]  IntegratorOutMax=[]  FilterOutMin=[]  FilterOutMax=[]  SumI1OutMin=[]  SumI1OutMax=[]  SumI2OutMin=[]  SumI2OutMax=[]  SumI3OutMin=[]  SumI3OutMax=[]  SumI4OutMin=[]  SumI4OutMax=[]  SumDOutMin=[]  SumDOutMax=[]  DifferentiatorOutMin=[]  DifferentiatorOutMax=[]  FilterDiffOutCoefMin=[]  FilterDiffOutCoefMax=[]  ReciprocalOutMin=[]  ReciprocalOutMax=[]  SumDenOutMin=[]  SumDenOutMax=[]  SumNumOutMin=[]  SumNumOutMax=[]  DivideOutMin=[]  DivideOutMax=[]  UdiffTsProdOutMin=[]  UdiffTsProdOutMax=[]  NTsProdOutMin=[]  NTsProdOutMax=[]  UintegralTsProdOutMin=[]  UintegralTsProdOutMax=[]  UngainTsProdOutMin=[]  UngainTsProdOutMax=[]  ClampingZeroOutDataTypeStr=Inherit: Inherit via back propagation  ClampingZeroOutMin=[]  ClampingZeroOutMax=[]  FilterDenConstantOutDataTypeStr=Inherit: Inherit via back propagation  FilterDenConstantOutMin=[]  FilterDenConstantOutMax=[]  PCopyOutDataTypeStr=Inherit: Inherit via back propagation  PCopyOutMin=[]  PCopyOutMax=[]  NCopyOutDataTypeStr=Inherit: Inherit via back propagation  NCopyOutMin=[]  NCopyOutMax=[]  IntegratorContinuousStateAttributes=''  IntegratorStateMustResolveToSignalObject=off  IntegratorRTWStateStorageClass=Auto  FilterContinuousStateAttributes=''  FilterStateMustResolveToSignalObject=off  FilterRTWStateStorageClass=Auto  ParallelPVariant=InternalParameters  IdealPVariant=Disabled  IVariant=InternalParameters  DVariant=InternalParameters  IntegratorVariant=Continuous  SatVariant=Enabled  AWVariant=BackCalculation  PCopyVariant=Disabled  TRVariant=Disabled  FdbkBlocksVariant=Forward  IdealPFdbkVariant=Disabled  SatFdbkVariant=Disabled  DerivativeFilterVariant=ContFilter  NVariant=InternalParameters  NCopyVariant=Disabled  FilterICVariant=InternalICsFilter  IntegratorICVariant=InternalICs  ExternalResetVariant=Disabled  TRSumVariant=Passthrough  SumFdbkVariant=Disabled  SumVariant=Sum_PID  TsampFilterVariant=InternalTs  TsampNgainVariant=Passthrough  TsampIntegralVariant=Disabled_SignalSpec  ExternalSaturationOutDataTypeStr=Inherit: Same as second input  DerivativeSourceVariant=ErrorSignal  PreIntVariant=InternalPreInt
  Sum : Sum  Inputs=|+-
  Sum1 : Sum  Inputs=|+-
  elev_cmd : Outport
  wires:
  Sum1/1 -> PID Controller/1
  Sum/1 -> elev_cmd/1
  Theta_ref/1 -> Sum1/1
  [q] -> Kq/1
  [theta] -> Sum1/2
  Kq/1 -> Sum/2
  PID Controller/1 -> Sum/1
  theta/1 -> [theta]
  q/1 -> [q]

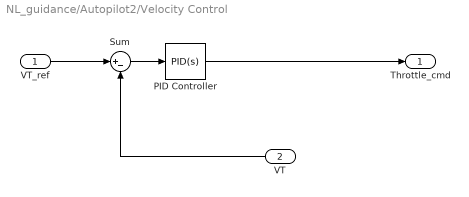
== system NL_guidance/Autopilot2/Velocity Control ==
  VT_ref : Inport
  VT : Inport  Port=2
  PID Controller : slpidlib/PID Controller  Controller=PID  Form=Parallel  TimeDomain=Continuous-time  UseExternalTs=off  SampleTime=-1  IntegratorMethod=Forward Euler  FilterMethod=Forward Euler  ControllerParametersSource=internal  P=C_vel.Kp  I=C_vel.Ki  UseKiTs=off  D=C_vel.Kd  UseExternalDerivativeSource=off  N=C_vel.N  UseFilter=on  TunerSelectOption=Transfer Function Based (PID Tuner App)  InitialConditionSource=internal  InitialConditionForIntegrator=0  InitialConditionForFilter=0  DifferentiatorICPrevScaledInput=0  ExternalReset=none  TrackingMode=off  Kt=1  LimitOutput=on  SatLimitsSource=internal  UpperSaturationLimit=0.51  LowerSaturationLimit=-0.49  LinearizeAsGain=on  AntiWindupMode=back-calculation  Kb=1  LimitIntegrator=off  UpperIntegratorSaturationLimit=inf  LowerIntegratorSaturationLimit=-inf  POutMin=[]  POutMax=[]  IOutMin=[]  IOutMax=[]  DOutMin=[]  DOutMax=[]  NOutMin=[]  NOutMax=[]  SumOutMin=[]  SumOutMax=[]  SaturationOutMin=[]  SaturationOutMax=[]  PParamMin=[]  PParamMax=[]  IParamMin=[]  IParamMax=[]  DParamMin=[]  DParamMax=[]  NParamMin=[]  NParamMax=[]  KbParamMin=[]  KbParamMax=[]  KtParamMin=[]  KtParamMax=[]  KbOutMin=[]  KbOutMax=[]  KtOutMin=[]  KtOutMax=[]  IntegratorOutMin=[]  IntegratorOutMax=[]  FilterOutMin=[]  FilterOutMax=[]  SumI1OutMin=[]  SumI1OutMax=[]  SumI2OutMin=[]  SumI2OutMax=[]  SumI3OutMin=[]  SumI3OutMax=[]  SumI4OutMin=[]  SumI4OutMax=[]  SumDOutMin=[]  SumDOutMax=[]  DifferentiatorOutMin=[]  DifferentiatorOutMax=[]  FilterDiffOutCoefMin=[]  FilterDiffOutCoefMax=[]  ReciprocalOutMin=[]  ReciprocalOutMax=[]  SumDenOutMin=[]  SumDenOutMax=[]  SumNumOutMin=[]  SumNumOutMax=[]  DivideOutMin=[]  DivideOutMax=[]  UdiffTsProdOutMin=[]  UdiffTsProdOutMax=[]  NTsProdOutMin=[]  NTsProdOutMax=[]  UintegralTsProdOutMin=[]  UintegralTsProdOutMax=[]  UngainTsProdOutMin=[]  UngainTsProdOutMax=[]  ClampingZeroOutDataTypeStr=Inherit: Inherit via back propagation  ClampingZeroOutMin=[]  ClampingZeroOutMax=[]  FilterDenConstantOutDataTypeStr=Inherit: Inherit via back propagation  FilterDenConstantOutMin=[]  FilterDenConstantOutMax=[]  PCopyOutDataTypeStr=Inherit: Inherit via back propagation  PCopyOutMin=[]  PCopyOutMax=[]  NCopyOutDataTypeStr=Inherit: Inherit via back propagation  NCopyOutMin=[]  NCopyOutMax=[]  IntegratorContinuousStateAttributes=''  IntegratorStateMustResolveToSignalObject=off  IntegratorRTWStateStorageClass=Auto  FilterContinuousStateAttributes=''  FilterStateMustResolveToSignalObject=off  FilterRTWStateStorageClass=Auto  ParallelPVariant=InternalParameters  IdealPVariant=Disabled  IVariant=InternalParameters  DVariant=InternalParameters  IntegratorVariant=Continuous  SatVariant=Enabled  AWVariant=BackCalculation  PCopyVariant=Disabled  TRVariant=Disabled  FdbkBlocksVariant=Forward  IdealPFdbkVariant=Disabled  SatFdbkVariant=Disabled  DerivativeFilterVariant=ContFilter  NVariant=InternalParameters  NCopyVariant=Disabled  FilterICVariant=InternalICsFilter  IntegratorICVariant=InternalICs  ExternalResetVariant=Disabled  TRSumVariant=Passthrough  SumFdbkVariant=Disabled  SumVariant=Sum_PID  TsampFilterVariant=InternalTs  TsampNgainVariant=Passthrough  TsampIntegralVariant=Disabled_SignalSpec  ExternalSaturationOutDataTypeStr=Inherit: Same as second input  DerivativeSourceVariant=ErrorSignal  PreIntVariant=InternalPreInt
  Sum : Sum  Inputs=|+-
  Throttle_cmd : Outport
  wires:
  VT/1 -> Sum/2
  PID Controller/1 -> Throttle_cmd/1
  VT_ref/1 -> Sum/1
  Sum/1 -> PID Controller/1

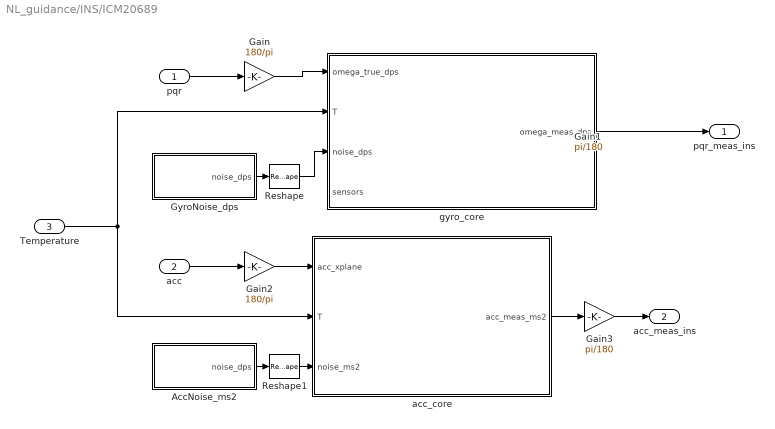
== system NL_guidance/INS/ICM20689 ==
  pqr : Inport
  acc : Inport  Port=2
  Temperature : Inport  Port=3
  AccNoise_ms2 : Subsystem
  Gain : Gain  Gain=180/pi
  Gain1 : Gain  Gain=pi/180
  Gain2 : Gain  Gain=180/pi
  Gain3 : Gain  Gain=pi/180
  GyroNoise_dps : Subsystem
  Reshape : Reshape  OutputDimensionality=Customize  OutputDimensions=[3 1]
  Reshape1 : Reshape  OutputDimensionality=Customize  OutputDimensions=[3 1]
  acc_core : MATLAB Function  TreatAsAtomicUnit=on
  gyro_core : MATLAB Function  TreatAsAtomicUnit=on
  pqr_meas_ins : Outport
  acc_meas_ins : Outport  Port=2
  wires:
  pqr/1 -> Gain/1
  Gain/1 -> gyro_core/1(omega_true_dps)
  Temperature/1 -> acc_core/2(T), gyro_core/2(T)
  acc/1 -> Gain2/1
  Gain2/1 -> acc_core/1(acc_xplane)
  acc_core/1(acc_meas_ms2) -> Gain3/1
  Gain3/1 -> acc_meas_ins/1
  GyroNoise_dps/1(noise_dps) -> Reshape/1
  Reshape/1 -> gyro_core/3(noise_dps)
  AccNoise_ms2/1(noise_dps) -> Reshape1/1
  Reshape1/1 -> acc_core/3(noise_ms2)
  gyro_core/1(omega_meas_dps) -> pqr_meas_ins/1

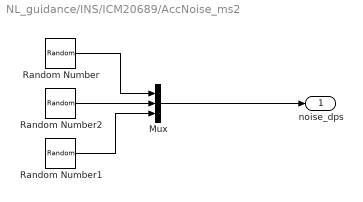
== system NL_guidance/INS/ICM20689/AccNoise_ms2 ==
  Mux : Mux  Inputs=3
  Random Number : RandomNumber  Variance=sensors.icm20689.acc.sigma_noise_ms2^2  Seed=sensors.seeds.icm20689.acc.noise(1)  SampleTime=sensors.sys.Ts
  Random Number1 : RandomNumber  Variance=sensors.icm20689.acc.sigma_noise_ms2^2  Seed=sensors.seeds.icm20689.acc.noise(3)  SampleTime=sensors.sys.Ts
  Random Number2 : RandomNumber  Variance=sensors.icm20689.acc.sigma_noise_ms2^2  Seed=sensors.seeds.icm20689.acc.noise(2)  SampleTime=sensors.sys.Ts
  noise_dps : Outport
  wires:
  Random Number/1 -> Mux/1
  Random Number2/1 -> Mux/2
  Random Number1/1 -> Mux/3
  Mux/1 -> noise_dps/1

== system NL_guidance/INS/ICM20689/GyroNoise_dps ==
  Mux : Mux  Inputs=3
  Random Number : RandomNumber  Variance=sensors.icm20689.gyro.sigma_noise_dps^2  Seed=sensors.seeds.icm20689.gyro.noise(1)  SampleTime=sensors.sys.Ts
  Random Number1 : RandomNumber  Variance=sensors.icm20689.gyro.sigma_noise_dps^2  Seed=sensors.seeds.icm20689.gyro.noise(3)  SampleTime=sensors.sys.Ts
  Random Number2 : RandomNumber  Variance=sensors.icm20689.gyro.sigma_noise_dps^2  Seed=sensors.seeds.icm20689.gyro.noise(2)  SampleTime=sensors.sys.Ts
  noise_dps : Outport
  wires:
  Random Number/1 -> Mux/1
  Random Number2/1 -> Mux/2
  Random Number1/1 -> Mux/3
  Mux/1 -> noise_dps/1

== matlab function NL_guidance/Xplane Interface/X-Plane Sensors ==
  settings: updateMethod=DISCRETE  sampleTime=0.05
  data: measurements output
function measurements = fcn()
%#codegen
coder.extrinsic('ins_read_xplane');

measurements = zeros(13,1);
tmp = zeros(1,13);

tmp = double(ins_read_xplane(0));
measurements(:) = tmp(:);

end

== matlab function NL_guidance/INS/ICM20689/gyro_core ==
  data: omega_meas_dps output double size=[3 1]; omega_true_dps input; T input; noise_dps input; sensors input
function omega_meas_dps = gyro_core(omega_true_dps, T, noise_dps, sensors)
%#codegen

coder.extrinsic('ins_gyro_errors_icm20689');
coder.extrinsic('evalin');
sensors = evalin('base', 'sensors');
omega_meas_dps = zeros(3,1);
tmp = zeros(3,1);
tmp = ins_gyro_errors_icm20689(omega_true_dps, T, noise_dps, sensors);

omega_meas_dps = tmp;
end

== matlab function NL_guidance/Autopilot2/Latero AutoPilotl/MATLAB Function ==
  data: psi_ref input; erro_psi output; psi_atual input
function erro_psi = calc_erro_proa(psi_ref, psi_atual)
    % Calcula a diferença simples
    diff = psi_ref - psi_atual;
    
    % Normaliza para o intervalo [-pi, +pi]
    % Isso garante que o avião sempre vire pelo lado mais curto.
    % Exemplo: Se quero ir para 350 mas estou em 10, o erro é -20, não +340.
    
    erro_psi = mod(diff + pi, 2*pi) - pi;
end

== matlab function NL_guidance/Autopilot2/MATLAB Function ==
  settings: updateMethod=DISCRETE
  data: pos_n input; psi_ref output; pos_e input; WPs input; R_accept input; h_ref output; v_ref output; wp_idx_monitor output; dist_monitor output; Xe_init input
function [psi_ref, h_ref, v_ref, wp_idx_monitor, dist_monitor] = Guidance_Star(pos_n, pos_e, WPs, R_accept, Xe_init)
    % Entradas:
    % pos_n, pos_e: Posição Atual em NED (m) [Inputs do Feedback]
    % WPs: Matriz de Waypoints [Norte, Leste, Altitude, Velocidade] [Parameter]
    % R_accept: Raio de aceitação (m) [Parameter]
    % Xe_init: Vetor de Estado Inicial 12x1 [Parameter]
    %          [u,v,w, p,q,r, phi,theta,psi, xN, xE, xD]
    
    % --- Inicialização Persistente ---
    persistent wp_idx
    
    if isempty(wp_idx)
        % Lógica de Inicialização no tempo t=0
        
        % 1. Definimos o primeiro alvo.
        % Se o avião já nasce no WP1 (conforme Xe), miramos no WP2.
        % Se o avião nasce longe de tudo, miramos no WP1 (opcional).
        wp_idx = 2; 
        
        % DICA: Aqui você poderia usar Xe_init para validar se o 
        % avião está onde o WP1 diz que deveria estar.
        % start_n = Xe_init(10);
        % start_e = Xe_init(11);
        % start_h = -Xe_init(12); % Conversão NED -> Altitude
    end
    
    % --- 1. Gestão de Missão (Troca de WP) ---
    num_wps = size(WPs, 1);
    
    % Proteção: Garante que o índice não exceda o número de WPs
    if wp_idx > num_wps
        wp_idx = num_wps;
    end
    
    % Define as coordenadas do Alvo Atual
    target_n = WPs(wp_idx, 1);
    target_e = WPs(wp_idx, 2);
    
    % Distância Euclidiana 2D até o alvo
    dist_error = sqrt((target_n - pos_n)^2 + (target_e - pos_e)^2);
    
    % Lógica de Troca:
    % Se (estou dentro do raio) E (NÃO é o último ponto) -> Próximo!
    if (dist_error <= R_accept) && (wp_idx < num_wps)
        wp_idx = wp_idx + 1;
    end
    
    % --- 2. Cálculo das Referências (Outputs) ---
    
    % Atualiza alvo (caso tenha trocado acima)
    target_n = WPs(wp_idx, 1);
    target_e = WPs(wp_idx, 2);
    
    % A. Heading Desejado (Line of Sight Puro)
    delta_n = target_n - pos_n;
    delta_e = target_e - pos_e;
    psi_ref = atan2(delta_e, delta_n); % Retorna [-pi, +pi]
    
    % B. Referências de Altitude e Velocidade
    % Nota: Aqui ocorre um degrau se a altitude atual for muito diferente
    % da altitude do WP alvo. O piloto automático deve suavizar isso.
    h_ref = WPs(wp_idx, 3);
    v_ref = WPs(wp_idx, 4);
    
    % --- 3. Saídas de Monitoramento ---
    wp_idx_monitor = wp_idx;
    dist_monitor = dist_error;
end

== matlab function NL_guidance/Xplane Interface/X-Plane Actuators ==
  settings: updateMethod=DISCRETE  sampleTime=0.05
  data: u input
function fcn(u)
%#codegen
coder.extrinsic('ins_send_xplane');
ins_send_xplane(u);
end

== matlab function NL_guidance/INS/ICM20689/acc_core ==
  data: acc_xplane input double size=[3 1]; T input double size=[1 1]; noise_ms2 input; acc_meas_ms2 output double size=[3 1]; sensors parameter
function acc_meas_ms2 = acc_core(acc_xplane, T, noise_ms2, sensors)
% Núcleo do modelo de erro do acelerômetro ICM20689.
% Entrada:
%   acc_xplane  : [3x1] aceleração de referência em m/s^2
%   T           : [1x1] temperatura em °C
%   noise_ms2   : [3x1] ruído externo em m/s^2
%   sensors     : struct com parâmetros dos sensores
% Saída:
%   acc_meas_ms2 : [3x1] aceleração medida em m/s^2

acc_xplane = acc_xplane(:);
noise_ms2  = noise_ms2(:);

acc = sensors.icm20689.acc;

% (1) Montagem nominal
roll = acc.roll_mount_deg*pi/180;
pit = acc.pitch_mount_deg*pi/180;
yaw = acc.yaw_mount_deg*pi/180;
R_roll = [1 0 0; 0 cos(roll) sin(roll);0 -sin(roll) cos(roll)];
R_pitch = [cos(pit) 0 -sin(pit); 0 1 0; sin(pit) 0 cos(pit)];
R_yaw = [ cos(yaw) sin(yaw) 0; -sin(yaw) cos(yaw) 0;0 0 1];
R_b2s = R_roll*R_pitch*R_yaw;
acc_nom = R_b2s * acc_xplane;
% (2) Misalignment
acc_misaligned = acc.R_mis * acc_nom;
% (3) Cross-axis
acc_cross = acc.Ca * acc_misaligned;
% (4) Scale factor com temperatura
sf = acc.sf_fixed + (T - acc.T_ref).*acc.k_sf;   % 1x3
acc_sf = acc_cross .* sf(:);

% (5) Não-linearidade
FS = acc.fundo_escala;  % m/s^2
acc_nl = acc_sf + (acc_sf.^3) .* (acc.k3(:) / (FS^2));
% (6) Bias com drift térmico
bias_g = acc.bias0_g + (T - acc.T_ref).*acc.kT_bias_g_per_C; % 1x3 em g
bias_ms2 = bias_g(:) * acc.gravity;
% (7) Soma com ruído externo
acc_ana = acc_nl + bias_ms2 + noise_ms2;
% (8) Saturação física
acc_sat = min(max(acc_ana, -acc.fundo_escala), acc.fundo_escala);
% (9) Quantização em LSB
acc_g = acc_sat / acc.gravity;
counts = round(acc_g * acc.sens_LSB_per_g);
counts = min(max(counts, -32768), 32767);
% (10) Zona morta em LSB
D = acc.deadzone_LSB;
abs_c = abs(counts);
counts_dz = zeros(size(counts));
mask = abs_c > D;
counts_dz(mask) = sign(counts(mask)) .* (abs_c(mask) - D);
% (11) Volta para m/s^2
acc_meas_g = counts_dz / acc.sens_LSB_per_g;
acc_meas_ms2 = acc_meas_g * acc.gravity;
end

== matlab function NL_guidance/INS/MATLAB Function ==
  data: acc_b_in input; euler_out output; gyro_b_in input; reset input; sample_valid input; t_now input; vel_out output; pos_out output; acc_n_out output; qb_out output
function [euler_out, vel_out, pos_out, acc_n_out, qb_out] = DBN_block( ...
    acc_b_in, gyro_b_in, reset, sample_valid, t_now)
%#codegen

coder.extrinsic('DBN_solver');
coder.extrinsic('evalin');

euler_out = zeros(3,1);
vel_out   = zeros(3,1);
pos_out   = zeros(3,1);
acc_n_out = zeros(3,1);
qb_out    = zeros(4,1);

DBN_params = evalin('base', 'DBN_params');

euler_tmp = zeros(3,1);
vel_tmp   = zeros(3,1);
pos_tmp   = zeros(3,1);
acc_tmp   = zeros(3,1);
qb_tmp    = zeros(4,1);

[euler_tmp, vel_tmp, pos_tmp, acc_tmp, qb_tmp] = DBN_solver( ...
    acc_b_in, gyro_b_in, reset, sample_valid, t_now, DBN_params);

euler_out = euler_tmp;
vel_out   = vel_tmp;
pos_out   = pos_tmp;
acc_n_out = acc_tmp;
qb_out    = qb_tmp;

end
